simulink model "teste"  (R2018a)
settings: Solver=VariableStepAuto  StartTime=0.0  StopTime=20  RelTol=1e-3
settings Model: Creator=Usuario  LastModifiedBy=crist
settings DataIOCC: ReturnWorkspaceOutputs=on
settings SFSimCC: SimUseLocalCustomCode=on
settings RTWCC: RTWUseLocalCustomCode=on

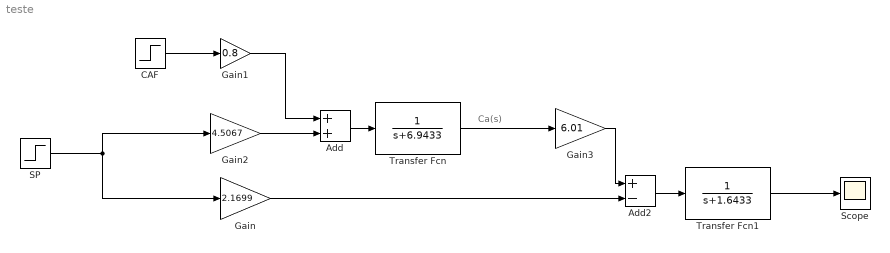
== system teste ==
  note: Ca(s)
  Add : Sum
  Add2 : Sum  Inputs=+-
  CAF : Step  Time=10  After=0  SampleTime=0.01
  Gain : Gain  Gain=2.1699
  Gain1 : Gain  Gain=0.8
  Gain2 : Gain  Gain=4.5067
  Gain3 : Gain  Gain=6.01
  SP : Step  Time=5  SampleTime=0.01
  Scope : Scope
  Transfer Fcn : TransferFcn  Denominator=[1 6.9433]
  Transfer Fcn1 : TransferFcn  Denominator=[1 1.6433]
  wires:
  SP/1 -> Gain/1, Gain2/1
  CAF/1 -> Gain1/1
  Add/1 -> Transfer Fcn/1
  Gain1/1 -> Add/1
  Gain2/1 -> Add/2
  Transfer Fcn/1 -> Gain3/1
  Gain3/1 -> Add2/1
  Gain/1 -> Add2/2
  Add2/1 -> Transfer Fcn1/1
  Transfer Fcn1/1 -> Scope/1
